simulink model "ConcatSingleTo64"  (R2024a)
settings: Solver=VariableStepAuto  StartTime=0.0  StopTime=1  RelTol=1e-3
libraries: hdlsllib x2
settings Model: Creator=acuadros  LastModifiedBy=acuadros
settings OptimizationCC: BlockReduction=off  ConditionallyExecuteInputs=off

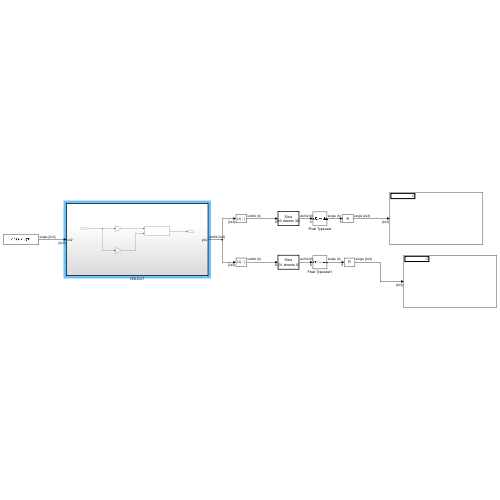
[thumbnail: Simulink's stored preview of the top-level diagram]
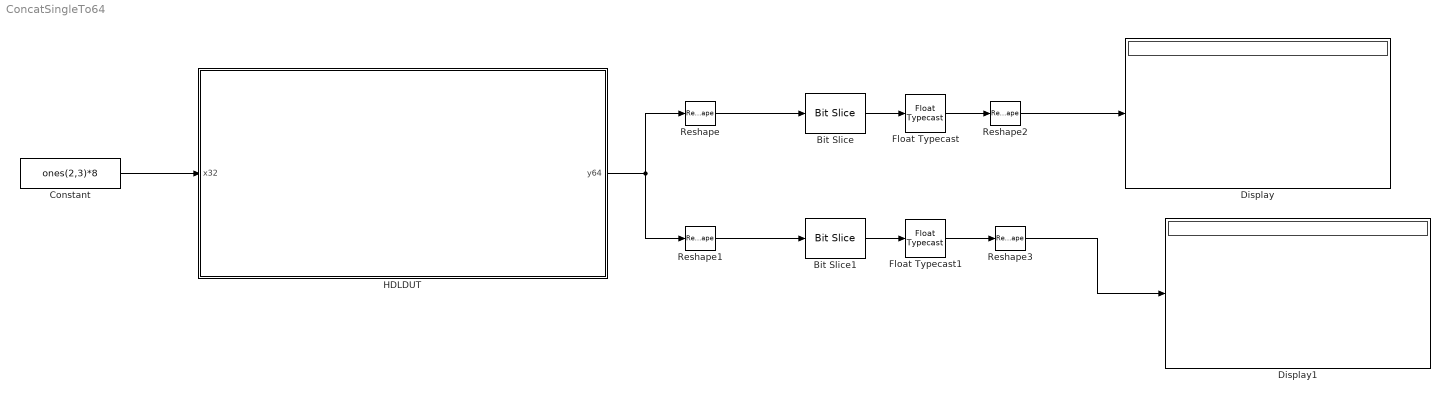
== system ConcatSingleTo64 ==
  Bit Slice : hdlsllib/Logic and Bit Operations/Bit Slice  lidx=63  ridx=32
  Bit Slice1 : hdlsllib/Logic and Bit Operations/Bit Slice  lidx=31  ridx=0
  Constant : Constant  Value=ones(2,3)*8  OutDataTypeStr=single  SampleTime=1
  Display : Display
  Display1 : Display
  Float Typecast : FloatTypecast
  Float Typecast1 : FloatTypecast
  HDLDUT : Subsystem  TreatAsAtomicUnit=on
  Reshape : Reshape
  Reshape1 : Reshape
  Reshape2 : Reshape  OutputDimensionality=Customize  OutputDimensions=[2,3]
  Reshape3 : Reshape  OutputDimensionality=Customize  OutputDimensions=[2,3]
  wires:
  Constant/1 -> HDLDUT/1(x32)
  HDLDUT/1(y64) -> Reshape1/1, Reshape/1
  Bit Slice/1 -> Float Typecast/1
  Float Typecast/1 -> Reshape2/1
  Bit Slice1/1 -> Float Typecast1/1
  Float Typecast1/1 -> Reshape3/1
  Reshape/1 -> Bit Slice/1
  Reshape1/1 -> Bit Slice1/1
  Reshape2/1 -> Display/1
  Reshape3/1 -> Display1/1

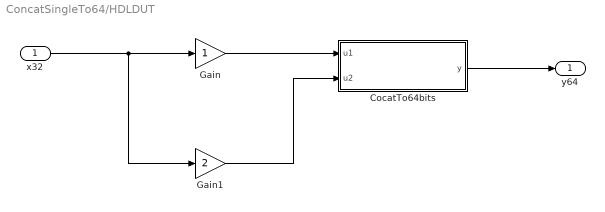
== system ConcatSingleTo64/HDLDUT ==
  x32 : Inport
  CocatTo64bits : MATLAB Function  TreatAsAtomicUnit=on
  Gain : Gain
  Gain1 : Gain  Gain=2
  y64 : Outport
  wires:
  Gain1/1 -> CocatTo64bits/2(u2)
  Gain/1 -> CocatTo64bits/1(u1)
  x32/1 -> Gain1/1, Gain/1
  CocatTo64bits/1(y) -> y64/1

== matlab function ConcatSingleTo64/HDLDUT/CocatTo64bits ==
  data: u1 input; y output; u2 input
function y = fcn(u1, u2)
% npu with a single element kernel 
y = hdl.npufun(@kernel, [1 1], u1, u2);

end

function out = kernel(in1, in2)
% use word2bits to get the bit representation of each input
a = hdl.word2bits(in1,32);
b = hdl.word2bits(in2,32);
% concatenate the bit vectors
out = bitconcat([a;b]);

end
